simulink model "LongitudinalControllerMPC"  (R2022a)
settings: Solver=VariableStepAuto  StartTime=0.0  StopTime=10.0  RelTol=1e-3
undefined symbols (not defined in the file): LongitudinalMPC_F, LongitudinalMPC_FeedbackGainKmpc, LongitudinalMPC_H, LongitudinalMPC_Nc, LongitudinalMPC_Np, LongitudinalMPC_Phi, LongitudinalMPC_PhiF, LongitudinalMPC_PhiR, LongitudinalMPC_ReferenceGainKy
libraries: CarMaker4SL x2
settings Model: Creator=krisz  LastModifiedBy=Krisztian

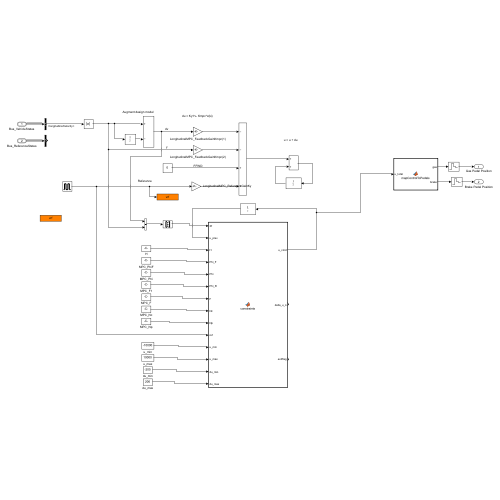
[thumbnail: Simulink's stored preview of the top-level diagram]
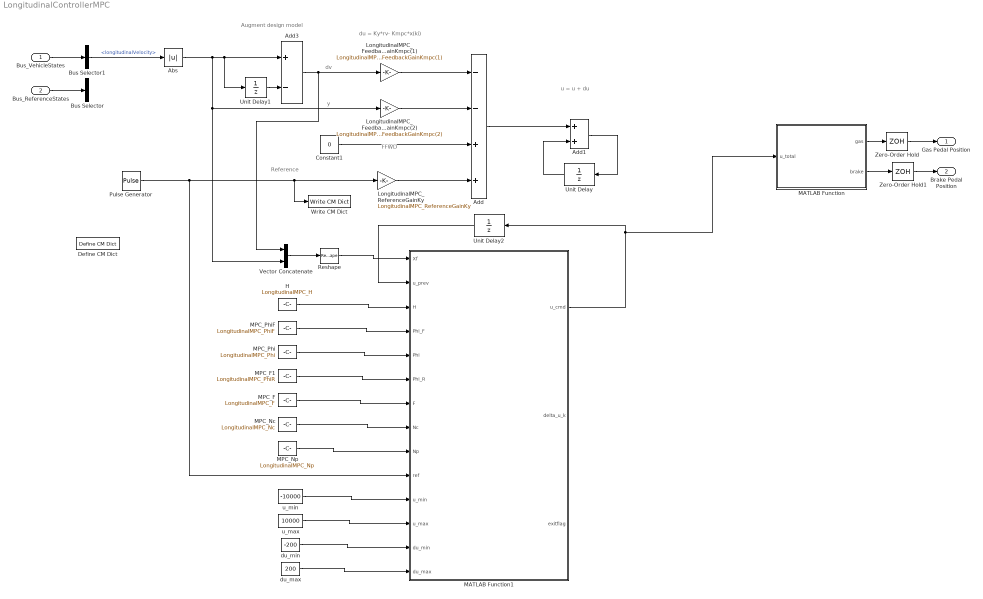
== system LongitudinalControllerMPC ==
  note: FFWD
  note: u = u + du
  note: du = Ky*rv- Kmpc*x(ki)
  note: Augment design model
  note: Reference
  note: dv
  note: y
  Bus_VehicleStates : Inport  OutDataTypeStr=Bus: bus_VehicleStates
  Bus_ReferenceStates : Inport  Port=2  OutDataTypeStr=Bus: bus_ReferenceStates
  Abs : Abs  SaturateOnIntegerOverflow=off
  Add : Sum  Inputs=--++
  Add1 : Sum
  Add3 : Sum  Inputs=+-
  Bus Selector : BusSelector  OutputSignals=referenceSpeed
  Bus Selector1 : BusSelector  OutputSignals=longitudinalVelocity
  Constant1 : Constant  Value=0
  Define CM Dict : CarMaker4SL/Define CM Dict  xname=vrf  xmono=off  xtype=Double4  xdvaplace=None  xnstates=0  xfirststate=0  xinitial=0
  H : Constant  Value=LongitudinalMPC_H
  LongitudinalMPC_FeedbackGainKmpc(1) : Gain  Gain=LongitudinalMPC_FeedbackGainKmpc(1)
  LongitudinalMPC_FeedbackGainKmpc(2) : Gain  Gain=LongitudinalMPC_FeedbackGainKmpc(2)
  LongitudinalMPC_ReferenceGainKy : Gain  Gain=LongitudinalMPC_ReferenceGainKy
  MATLAB Function : MATLAB Function  TreatAsAtomicUnit=on
  MATLAB Function1 : MATLAB Function  TreatAsAtomicUnit=on
  MPC_F : Constant  Value=LongitudinalMPC_F
  MPC_F1 : Constant  Value=LongitudinalMPC_PhiR
  MPC_Nc : Constant  Value=LongitudinalMPC_Nc
  MPC_Np : Constant  Value=LongitudinalMPC_Np
  MPC_Phi : Constant  Value=LongitudinalMPC_Phi  VectorParams1D=off
  MPC_PhiF : Constant  Value=LongitudinalMPC_PhiF
  Pulse Generator : DiscretePulseGenerator  PulseType=Time based  Amplitude=15  Period=60  PulseWidth=70
  Reshape : Reshape  OutputDimensionality=Column vector (2-D)
  Unit Delay : UnitDelay  SampleTime=-1  HasFrameUpgradeWarning=on
  Unit Delay1 : UnitDelay  SampleTime=-1  HasFrameUpgradeWarning=on
  Unit Delay2 : UnitDelay  SampleTime=-1  HasFrameUpgradeWarning=on
  Vector Concatenate : Concatenate
  Write CM Dict : CarMaker4SL/Write CM Dict  xname=vrf  xsync=off
  Zero-Order Hold : ZeroOrderHold  SampleTime=-1
  Zero-Order Hold1 : ZeroOrderHold  SampleTime=-1
  du_max : Constant  Value=200
  du_min : Constant  Value=-200
  u_max : Constant  Value=10000
  u_min : Constant  Value=-10000  VectorParams1D=off
  Gas Pedal Position : Outport
  Brake Pedal Position : Outport  Port=2
  wires:
  Bus_ReferenceStates/1 -> Bus Selector/1
  Bus_VehicleStates/1 -> Bus Selector1/1
  LongitudinalMPC_FeedbackGainKmpc(1)/1 -> Add/1
  Add3/1 -> Vector Concatenate/1, LongitudinalMPC_FeedbackGainKmpc(1)/1
  Add1/1 -> Unit Delay/1
  Unit Delay/1 -> Add1/2
  Abs/1 -> LongitudinalMPC_FeedbackGainKmpc(2)/1, Vector Concatenate/2, Unit Delay1/1, Add3/1
  LongitudinalMPC_FeedbackGainKmpc(2)/1 -> Add/2
  Bus Selector1/1 -> Abs/1  "<longitudinalVelocity>"
  Unit Delay1/1 -> Add3/2
  LongitudinalMPC_ReferenceGainKy/1 -> Add/4
  MATLAB Function/1(gas) -> Zero-Order Hold/1
  MATLAB Function/2(brake) -> Zero-Order Hold1/1
  Pulse Generator/1 -> MATLAB Function1/10(ref), LongitudinalMPC_ReferenceGainKy/1, Write CM Dict/1
  Zero-Order Hold/1 -> Gas Pedal Position/1
  Zero-Order Hold1/1 -> Brake Pedal Position/1
  Constant1/1 -> Add/3
  Add/1 -> Add1/1
  du_max/1 -> MATLAB Function1/14(du_max)
  du_min/1 -> MATLAB Function1/13(du_min)
  MPC_PhiF/1 -> MATLAB Function1/4(Phi_F)
  MPC_Nc/1 -> MATLAB Function1/8(Nc)
  H/1 -> MATLAB Function1/3(H)
  MPC_Phi/1 -> MATLAB Function1/5(Phi)
  MPC_F/1 -> MATLAB Function1/7(F)
  u_min/1 -> MATLAB Function1/11(u_min)
  MPC_Np/1 -> MATLAB Function1/9(Np)
  u_max/1 -> MATLAB Function1/12(u_max)
  Unit Delay2/1 -> MATLAB Function1/2(u_prev)
  Reshape/1 -> MATLAB Function1/1(Xf)
  Vector Concatenate/1 -> Reshape/1
  MPC_F1/1 -> MATLAB Function1/6(Phi_R)
  MATLAB Function1/1(u_cmd) -> Unit Delay2/1, MATLAB Function/1(u_total)

== matlab function LongitudinalControllerMPC/MATLAB Function1 ==
  data: Xf input; u_cmd output; u_prev input; H input; Phi_F input; Phi input; Phi_R input; F input; Nc input; Np input; ref input; u_min input; u_max input; du_min input; du_max input; delta_u_k output; exitflag output
function [u_cmd, delta_u_k, exitflag] = constraints( ...
    Xf, u_prev, ...
    H, Phi_F, Phi, Phi_R, F, ...
    Nc, Np, ref,  ...
    u_min, u_max, du_min, du_max)

    C1 = ones(Nc, 1);
    C2 = kron(tril(ones(Nc)), 1);

    Umax = ones(Nc, 1) * u_max;
    Umin = ones(Nc, 1) * u_min;
    dUmax = ones(Nc, 1) * du_max;
    dUmin = ones(Nc, 1) * du_min;
    %Ymax = ones(Np, 1) * y_max;
    %Ymin = ones(Np, 1) * y_min;

    M1 = [-C2; C2];
    M2 = [-eye(Nc); eye(Nc)];
    %M3 = [-Phi; Phi];
    M = [M1; M2];

    N1 = [-Umin + C1 * u_prev; Umax - C1 * u_prev];
    N2 = [-dUmin; dUmax];
    % N3 = [-Ymin + F * Xf; Ymax - F * Xf];
    gamma = [N1; N2];

    f = -(Phi_R * ref - Phi_F * Xf);

    deltaU = QPhild(H, f, M, gamma);

    if all(M * deltaU <= gamma)
        exitflag = 1;
    else
        exitflag = 0;
    end

    delta_u_k = deltaU(1:1);
    delta_u_k = min(max(delta_u_k, du_min), du_max);
    u_cmd = u_prev + delta_u_k;
    u_cmd = min(max(u_cmd, u_min), u_max);
end

function eta = QPhild(H, f, A_cons, b)
%QPHILD Hildreth QP algorithm pasted for MATLAB Function block usage.

    [n1, ~] = size(A_cons);
    eta = -H \ f;
    kk = 0;

    for i = 1:n1
        if A_cons(i, :) * eta > b(i)
            kk = kk + 1;
        end
    end

    if kk == 0
        return;
    end

    P = A_cons * (H \ A_cons');
    d = (A_cons * (H \ f) + b);
    [n, m] = size(d);
    x_ini = zeros(n, m);
    lambda = x_ini;

    for km = 1:38
        lambda_p = lambda;
        for i = 1:n
            w = P(i, :) * lambda - P(i, i) * lambda(i, 1);
            w = w + d(i, 1);
            la = -w / P(i, i);
            lambda(i, 1) = max(0, la);
        end

        al = (lambda - lambda_p)' * (lambda - lambda_p);
        if al < 1e-7
            break;
        end
    end

    eta = -H \ f - H \ A_cons' * lambda;
end

== matlab function LongitudinalControllerMPC/MATLAB Function ==
  data: u_total input; gas output; brake output
function [gas, brake] = mapControlToPedals(u_total)
    % MAPCONTROLTOPEDALS Szétválasztja a szabályozó jelét gáz- és fékpedálra.
    %
    % Bemenetek:
    %   u_total  - A szabályozó által számított teljes erő [N]
    %   u_max    - A rendszer maximális ereje (skálázási alap) [N]
    %   deadband - Holtsáv (opcionális, pl. 0.01 a 1%-os sávhoz)
    

    % 1. Normalizálás [-1, 1] tartományba
    u_norm = u_total/10000 ;
    
    % Korlátozás a biztonság kedvéért
    %u_norm = max(-1, min(1, u_norm));

    % 2. Holtsáv alkalmazása a rángatás elkerülésére

    % 3. Szétválasztás (Gas: 0..1, Brake: 0..1)
    if u_norm >= 0
        gas   = u_norm;
        brake = 0;
    else
        gas   = 0;
        brake = abs(u_norm); % A fékjel is pozitív elmozdulás/nyomás
    end
end
